simulink model "KALMAN_FILTER"  (R2016b)
settings: Solver=VariableStepAuto  StartTime=0.0  StopTime=10.0  RelTol=1e-3
settings Model: Creator=liana  LastModifiedBy=liana

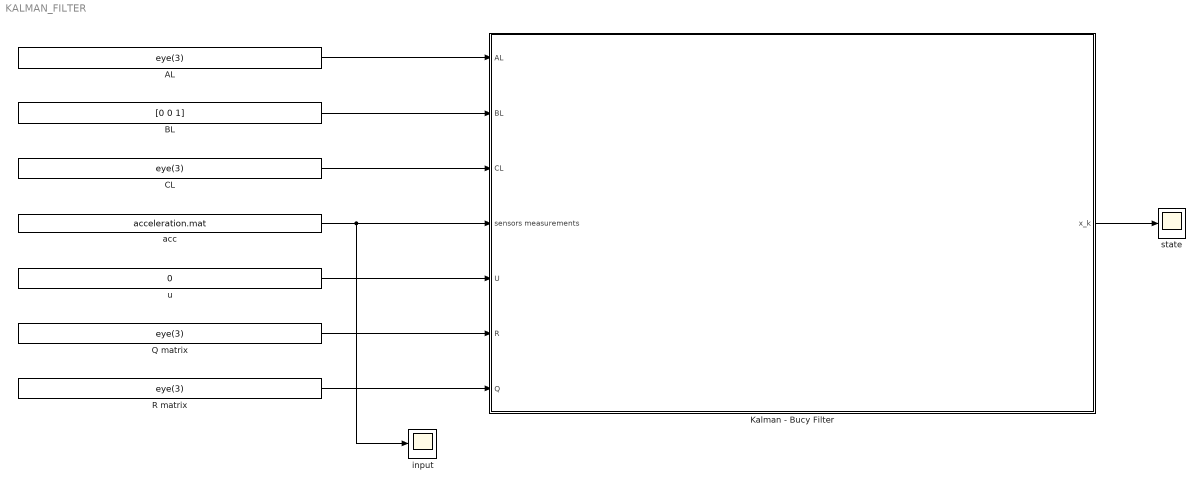
== system KALMAN_FILTER ==
  AL : Constant  Value=eye(3)
  BL : Constant  Value=[0 0 1]
  CL : Constant  Value=eye(3)
  Kalman - Bucy Filter : Subsystem
  Q matrix : Constant  Value=eye(3)
  R matrix : Constant  Value=eye(3)
  acc : FromFile  FileName=acceleration.mat  SampleTime=0
  input : Scope
  state : Scope
  u : Constant  Value=0
  wires:
  Q matrix/1 -> Kalman - Bucy Filter/6(R)
  R matrix/1 -> Kalman - Bucy Filter/7(Q)
  AL/1 -> Kalman - Bucy Filter/1(AL)
  CL/1 -> Kalman - Bucy Filter/3(CL)
  BL/1 -> Kalman - Bucy Filter/2(BL)
  Kalman - Bucy Filter/1(x_k) -> state/1
  u/1 -> Kalman - Bucy Filter/5(U)
  acc/1 -> input/1, Kalman - Bucy Filter/4(sensors measurements)

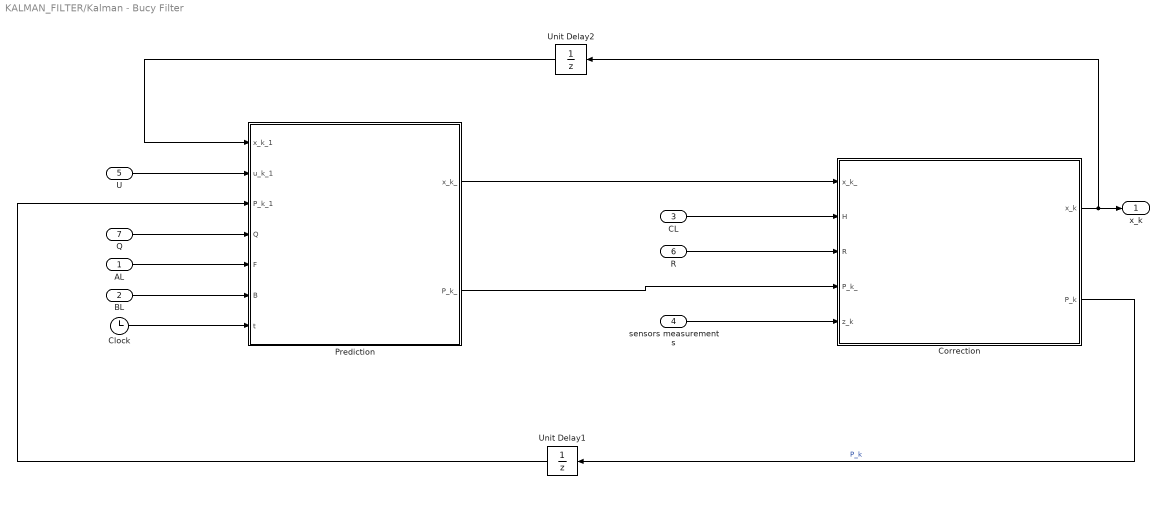
== system KALMAN_FILTER/Kalman - Bucy Filter ==
  AL : Inport
  BL : Inport  Port=2
  CL : Inport  Port=3
  sensors measurements : Inport  Port=4
  U : Inport  Port=5
  R : Inport  Port=6
  Q : Inport  Port=7
  Clock : Clock
  Correction : MATLAB Function  TreatAsAtomicUnit=on
  Prediction : MATLAB Function  TreatAsAtomicUnit=on
  Unit Delay1 : UnitDelay  SampleTime=-1
  Unit Delay2 : UnitDelay  SampleTime=-1
  x_k : Outport
  wires:
  Prediction/2(P_k_) -> Correction/4(P_k_)
  Prediction/1(x_k_) -> Correction/1(x_k_)
  AL/1 -> Prediction/5(F)
  CL/1 -> Correction/2(H)
  Clock/1 -> Prediction/7(t)
  Q/1 -> Prediction/4(Q)
  sensors measurements/1 -> Correction/5(z_k)
  BL/1 -> Prediction/6(B)
  U/1 -> Prediction/2(u_k_1)
  R/1 -> Correction/3(R)
  Correction/2(P_k) -> Unit Delay1/1  "P_k"
  Correction/1(x_k) -> Unit Delay2/1, x_k/1
  Unit Delay1/1 -> Prediction/3(P_k_1)
  Unit Delay2/1 -> Prediction/1(x_k_1)

== matlab function KALMAN_FILTER/Kalman - Bucy Filter/Prediction ==
  data: x_k_1 input size=[3, 1]; x_k_ output; u_k_1 input; P_k_1 input size=[3,3]; Q input; F input; B input; P_k_ output; t input
function [x_k_, P_k_] = prediction(x_k_1, u_k_1, P_k_1, Q, F,B, t)

    % initial value 
    if t == 0
        x_k_1 = zeros(3,1);
        P_k_1 = eye(3);
    end

    x_k_ = F * x_k_1 + B * u_k_1';
    P_k_ = F * P_k_1 * F' + Q;
    

end

== matlab function KALMAN_FILTER/Kalman - Bucy Filter/Correction ==
  data: x_k_ input; H input; R input; P_k_ input; z_k input; x_k output; P_k output
function [x_k, P_k]  = correction(x_k_ , H, R, P_k_ ,z_k)

    n = size(P_k_);
    I = eye(n);

    K_k = P_k_ * H' * pinv(H * P_k_ * H' + R);
    
    x_k = x_k_ + K_k * (z_k - H * x_k_);
    
    P_k = ( I - K_k * H) * P_k_;

end
